simulink model "Part1_1"  (R2017a)
settings: Solver=VariableStepAuto  StartTime=0.0  StopTime=10.0  RelTol=1e-3
libraries: dspquant2 x2, dsparch4 x1, dspsigops x1
settings Model: Creator=mhuynh7  LastModifiedBy=mhuynh7

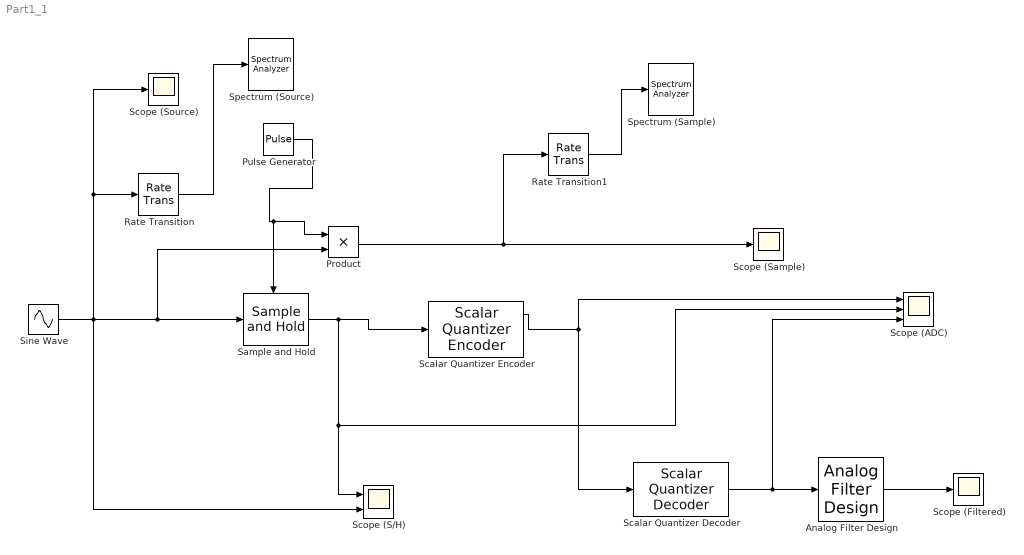
== system Part1_1 ==
  Analog Filter Design : dsparch4/Analog Filter Design  method=Butterworth  filttype=Lowpass  N=20  Wlo=1000*pi  Whi=80  Rp=2  Rs=40
  Product : Product
  Pulse Generator : DiscretePulseGenerator  PulseType=Time based  Period=0.001/8  PulseWidth=50
  Rate Transition : RateTransition  OutPortSampleTime=1e-5
  Rate Transition1 : RateTransition  OutPortSampleTime=1e-5
  Sample and Hold : dspsigops/Sample and Hold  trig=Rising edge  initCond=0  latchinput=off
  Scalar Quantizer Decoder : dspquant2/Scalar Quantizer Decoder  invalidin=Clip  CBsource=Specify via dialog  codebook=[-1.75:0.5:1.75]  dataType=double  isSigned=on  wordLen=16  udDataType=sfix(16)  fracBitsMode=Best precision  numFracBits=11  OutDataTypeStr=double  LastOutDataTypeStr=double
      settings: SourceProductName=DSP System Toolbox  SourceProductBaseCode=DS
  Scalar Quantizer Encoder : dspquant2/Scalar Quantizer Encoder  paramSrc=Specify via dialog  partType=Bounded  BBoundary=[-2:0.5:2]  UBoundary=[2:9]  SearchMethod=Linear  tieBreakRule=Choose the lower index  outQU=on  outQError=off  codebook=[-1.75:0.5:1.75]  outStatus=off  invalidin=Clip  idtype=int32  roundingMode=Floor  overflowMode=off
      settings: SourceProductName=DSP System Toolbox  SourceProductBaseCode=DS
  Scope (ADC) : Scope  NumInputPorts=3
  Scope (Filtered) : Scope
  Scope (S/H) : Scope  NumInputPorts=2
  Scope (Sample) : Scope
  Scope (Source) : Scope
  Sine Wave : Sin  Amplitude=2  Frequency=1000*pi  SampleTime=0
  Spectrum (Sample) : SpectrumAnalyzer
  Spectrum (Source) : SpectrumAnalyzer
  wires:
  Sine Wave/1 -> Scope (S/H)/2, Product/2, Sample and Hold/1, Scope (Source)/1, Rate Transition/1
  Rate Transition/1 -> Spectrum (Source)/1
  Pulse Generator/1 -> Product/1, Sample and Hold/Trigger
  Product/1 -> Rate Transition1/1, Scope (Sample)/1
  Rate Transition1/1 -> Spectrum (Sample)/1
  Sample and Hold/1 -> Scope (ADC)/2, Scope (S/H)/1, Scalar Quantizer Encoder/1
  Scalar Quantizer Encoder/1 -> Scalar Quantizer Decoder/1, Scope (ADC)/1
  Scalar Quantizer Decoder/1 -> Scope (ADC)/3, Analog Filter Design/1
  Analog Filter Design/1 -> Scope (Filtered)/1
